simulink model "PVHome"  (R2022b)
settings: Solver=FixedStepDiscrete  StartTime=0.0  StopTime=2  FixedStep=5e-6  RelTol=1e-3
undefined symbols (not defined in the file): Ion, Lithium
libraries: spsSeriesRLCBranchLib x175, spsBreakerLib x103, spsPWMGeneratorDCDCLib x94, spsThyristorLib x78, slpidlib x72, spsIGBTDiodeLib x62, spsThreePhaseVIMeasurementLib x59, spsThreePhaseBreakerLib x45, spsVoltageMeasurementLib x45, spsDiodeLib x39, spsThreePhaseParallelRLCBranchLib x38, spsMosfetLib x32
(part 14 of 16)

== matlab function PVHome/Subsystem2/Centralized System ==
  data: H1_Pv_Breaker output; P_Pv input; Bi_B_Charge_Breaker_Buck output; Bi_B_Charge_Breaker_Boost output; H1_Grid_Breaker output; H1_Grid_Circuit_Breaker output; P_load input; Bi_B_Breaker_Discharge_Boost output; Bi_B_Breaker_Discharge_Buck output; H1_B_Ground_Discharge output; SOCbH1 input; Grid_Energy_Trading_Breaker output; Wind_Breaker_Boost output; P_Wind input; P_Real_Grid input; Wind_Breaker_Buck output; V_PV_1 input; V_Wind input; Wind_Power_Battery_Breaker_Boost output; Wind_Power_Battery_Breaker_Buck output; Battery_Passing_Voltage input; P_PV_2 input; V_PV_2 input; PV_2_Buck_Breaker output; PV_2_Boost_Breaker output
function [H1_Pv_Breaker, Bi_B_Charge_Breaker_Buck,Bi_B_Charge_Breaker_Boost, H1_Grid_Breaker, H1_Grid_Circuit_Breaker,Bi_B_Breaker_Discharge_Boost, Bi_B_Breaker_Discharge_Buck, H1_B_Ground_Discharge, Grid_Energy_Trading_Breaker, Wind_Breaker_Boost, Wind_Breaker_Buck, Wind_Power_Battery_Breaker_Boost, Wind_Power_Battery_Breaker_Buck, PV_2_Buck_Breaker, PV_2_Boost_Breaker] = control_logic(P_Pv, P_load, SOCbH1, P_Wind, P_Real_Grid, V_PV_1, V_Wind, Battery_Passing_Voltage, P_PV_2, V_PV_2)

% Make positive
P_Pv   = abs(P_Pv);
P_load = abs(P_load);
SOCbH1 = abs(SOCbH1);
P_Wind = abs(P_Wind);
V_PV_1 = abs(V_PV_1);
V_Wind = abs(V_Wind);
Battery_Passing_Voltage = abs(Battery_Passing_Voltage);
P_PV_2 = abs(P_PV_2);
V_PV_2 = abs(V_PV_2);

eps = 1;

%% DEFAULT STATES

% DC Ideal Switches (1 = ON) gets closed and power flows when 1
H1_Pv_Breaker = 0;
Bi_B_Charge_Breaker_Buck  = 0;
Bi_B_Charge_Breaker_Boost=0;
Bi_B_Breaker_Discharge_Boost=0;
Bi_B_Breaker_Discharge_Buck=0;
H1_B_Ground_Discharge=0;
Wind_Breaker_Boost=0;
Wind_Breaker_Buck=0;
Wind_Power_Battery_Breaker_Boost=0;
Wind_Power_Battery_Breaker_Buck=0;
PV_2_Buck_Breaker=0;
PV_2_Boost_Breaker=0;

% AC Breakers (0 = CLOSED) gets closed and power flows when 0
H1_Grid_Breaker = 1;  % default OPEN
H1_Grid_Circuit_Breaker = 1;  % default OPEN
Grid_Energy_Trading_Breaker=1; % default open



%% CASE 1: No PV and no Wind
if (P_Pv + P_Wind + P_PV_2) <= eps %eps=0.01 (almost 0)

    % DC OFF
    H1_Pv_Breaker = 0;
    Bi_B_Charge_Breaker_Buck  = 0;
    Bi_B_Breaker_Discharge_Boost=0;
    H1_B_Ground_Discharge=0;
    Bi_B_Breaker_Discharge_Buck=0;
    Wind_Breaker_Boost=0;
    Wind_Breaker_Buck=0;
    Wind_Power_Battery_Breaker_Boost=0;
    Wind_Power_Battery_Breaker_Buck=0;
    PV_2_Boost_Breaker=0;


    % AC CLOSED (use grid)
    H1_Grid_Breaker         = 0;
    H1_Grid_Circuit_Breaker = 1;
    Grid_Energy_Trading_Breaker=1; %energy trading window open


%% CASE 2: PV and wind > Load
elseif (P_Pv + P_Wind + P_PV_2) > P_load

    % Use PV
    H1_Pv_Breaker = 1;
    H1_Grid_Breaker = 1;
    H1_Grid_Circuit_Breaker = 1;

    if (SOCbH1) < 90 % if the value of soc is between is less than 90%, the battery can charge
        
        Bi_B_Breaker_Discharge_Boost=0;
        Bi_B_Breaker_Discharge_Buck=0;
        H1_B_Ground_Discharge=0;
        Grid_Energy_Trading_Breaker=1;
        

        if (V_PV_1 > V_Wind) %boosts up
            Wind_Power_Battery_Breaker_Boost=1;
            Wind_Power_Battery_Breaker_Buck=0;
            Wind_Breaker_Boost=1;
            Wind_Breaker_Buck=0;
            if (Battery_Passing_Voltage)>60
                Bi_B_Charge_Breaker_Buck=1;
                Bi_B_Charge_Breaker_Boost=0;
            elseif (Battery_Passing_Voltage<60)
                Bi_B_Charge_Breaker_Buck=0;
                Bi_B_Charge_Breaker_Boost=1;
            end

        elseif (V_PV_1 < V_Wind)
            Wind_Power_Battery_Breaker_Boost=0;
            Wind_Power_Battery_Breaker_Buck=1;
            Wind_Breaker_Boost=0;
            Wind_Breaker_Buck=1;
        
            if (Battery_Passing_Voltage)>60
                Bi_B_Charge_Breaker_Buck=1;
                Bi_B_Charge_Breaker_Boost=0;
            elseif (Battery_Passing_Voltage)<60
                Bi_B_Charge_Breaker_Buck=0;
                Bi_B_Charge_Breaker_Boost=1;
            end

        
        end 

        elseif (V_PV_2>V_PV_1)
            PV_2_Buck_Breaker=1;
            PV_2_Boost_Breaker=0;
        elseif (V_PV_2<V_PV_1)
            PV_2_Buck_Breaker=0;
            PV_2_Boost_Breaker=1;

        elseif SOCbH1==90
            Bi_B_Charge_Breaker_Boost=0;
            Bi_B_Charge_Breaker_Buck = 0;
            Bi_B_Breaker_Discharge_Boost=0;
            Bi_B_Breaker_Discharge_Buck=0;
            H1_B_Ground_Discharge=0;
            Grid_Energy_Trading_Breaker=0; %the power is sold to grid
        end


%% CASE 3: PV and wind < Load
elseif (P_Pv + P_Wind + P_PV_2) < (P_load) && (H1_Grid_Breaker~=0) %open (1 means open)

    % Use PV
    H1_Pv_Breaker = 1;
    H1_Grid_Circuit_Breaker = 0;
    Grid_Energy_Trading_Breaker=1;      
    Bi_B_Charge_Breaker_Buck=0; %no charging
    Bi_B_Charge_Breaker_Boost=0; %no charging

    if (V_PV_2>V_PV_1)
        PV_2_Buck_Breaker=1;
        PV_2_Boost_Breaker=0;
    elseif (V_PV_2<V_PV_1)
         PV_2_Buck_Breaker=0;
         PV_2_Boost_Breaker=1;
    end

    if (V_PV_1)>60
        Bi_B_Breaker_Discharge_Boost=1;
        Bi_B_Breaker_Discharge_Buck=0;
        H1_B_Ground_Discharge=1;
    elseif(V_PV_1)<60
        Bi_B_Breaker_Discharge_Boost=0;
        Bi_B_Breaker_Discharge_Buck=1;
        H1_B_Ground_Discharge=1;
    end

    if (V_PV_1 > V_Wind) %boosts up
        Wind_Power_Battery_Breaker_Boost=1;
        Wind_Power_Battery_Breaker_Buck=0;
        Wind_Breaker_Boost=1;
        Wind_Breaker_Buck=0;
        
    elseif (V_PV_1 < V_Wind)
        Wind_Power_Battery_Breaker_Boost=0;
        Wind_Power_Battery_Breaker_Buck=1;
        Wind_Breaker_Boost=0;
        Wind_Breaker_Buck=1;
    end 

    
   

           
%% CASE 4:
elseif (P_Pv + P_Wind + P_PV_2) < (P_load) && (H1_Grid_Breaker~=1) %closed (0) (no charging)

        % Use PV
    H1_Pv_Breaker = 1;
    H1_Grid_Circuit_Breaker = 0;
    Grid_Energy_Trading_Breaker=1;      
    Bi_B_Charge_Breaker_Buck=0; %(no charging)
    Bi_B_Charge_Breaker_Boost=0; %(no charging)
    Bi_B_Breaker_Discharge_Boost=0; %(no discharging also)
    Bi_B_Breaker_Discharge_Buck=0; %(no discharging also)
    H1_B_Ground_Discharge=0;

    if (V_PV_2>V_PV_1)
        PV_2_Buck_Breaker=1;
        PV_2_Boost_Breaker=0;
    elseif (V_PV_2<V_PV_1)
         PV_2_Buck_Breaker=0;
         PV_2_Boost_Breaker=1;
    end


    if (V_PV_1 > V_Wind) %boosts up
        Wind_Power_Battery_Breaker_Boost=1;
        Wind_Power_Battery_Breaker_Buck=0;
        Wind_Breaker_Boost=1;
        Wind_Breaker_Buck=0;
        
    elseif (V_PV_1 < V_Wind)
        Wind_Power_Battery_Breaker_Boost=0;
        Wind_Power_Battery_Breaker_Buck=1;
        Wind_Breaker_Boost=0;
        Wind_Breaker_Buck=1;
    end 


%% CASE 5:
elseif (P_Pv + P_Wind+ P_Real_Grid + P_PV_2) < P_Load 
    % Use PV
    H1_Grid_Breaker=0;
    H1_Pv_Breaker = 1;
    H1_Grid_Circuit_Breaker = 0;
    Grid_Energy_Trading_Breaker=1;      
    Bi_B_Charge_Breaker_Buck=0; %(no charging)
    Bi_B_Charge_Breaker_Boost=0; %(no charging)



    %discharging
    if (V_PV_1)>60
        Bi_B_Breaker_Discharge_Boost=1;
        Bi_B_Breaker_Discharge_Buck=0;
        H1_B_Ground_Discharge=1;
    elseif(V_PV_1)<60
        Bi_B_Breaker_Discharge_Boost=0;
        Bi_B_Breaker_Discharge_Buck=1;
        H1_B_Ground_Discharge=1;
    end

    if (V_PV_2>V_PV_1)
        PV_2_Buck_Breaker=1;
        PV_2_Boost_Breaker=0;
    elseif (V_PV_2<V_PV_1)
         PV_2_Buck_Breaker=0;
         PV_2_Boost_Breaker=1;
    end

    if (V_PV_1 > V_Wind) %boosts up
        Wind_Power_Battery_Breaker_Boost=1;
        Wind_Power_Battery_Breaker_Buck=0;
        Wind_Breaker_Boost=1;
        Wind_Breaker_Buck=0;
        
    elseif (V_PV_1 < V_Wind) %bucks down
        Wind_Power_Battery_Breaker_Boost=0;
        Wind_Power_Battery_Breaker_Buck=1;
        Wind_Breaker_Boost=0;
        Wind_Breaker_Buck=1;
    end 

end


end

== matlab function PVHome/Subsystem2/MATLAB Function ==
  data: V_PV input; duty output; I_PV input; deltaD input
function duty = mppt_pno(V_PV, I_PV, deltaD)

persistent prevP prevDuty

if isempty(prevP)
    prevP = 0;
    prevDuty = 0.5;   % Start at 50%
end

% Current PV power
P = V_PV * I_PV;

% Basic P&O
if P > prevP
    prevDuty = prevDuty + deltaD;
else
    prevDuty = prevDuty - deltaD;
end

% Safe duty limits for boost converter
if prevDuty > 0.75
    prevDuty = 0.75;
elseif prevDuty < 0.10
    prevDuty = 0.10;
end

% Update previous power
prevP = P;

% Output duty
duty = prevDuty;

end

== matlab function PVHome/Subsystem2/MATLAB Function1 ==
  data: u input
function export_live_data(u)
% export_live_data  MATLAB Function block that writes 4 signals live into Excel
% Input: u (4-element vector)
% Exact workbook path used: 'V:\IEEE\LIVEdata.xlsx'
%
% Structure preserved: all COM/workspace actions run via evalin('base', ...)

    coder.extrinsic('evalin','assignin','actxserver','datetime','char','warning');

    persistent initialized
    if isempty(initialized)
        initialized = false;
    end

    % Convert inputs to doubles
    a = double(u(1)); b = double(u(2)); c = double(u(3)); d = double(u(4));

    % Use an .xlsx workbook for live UI updates
    excelPath = 'V:\IEEE\LIVEdata.csv';

    % Initialization block executed once (all logic runs inside evalin strings)
    if ~initialized
        % Ensure Excel COM server exists in base workspace and open/create workbook
        evalin('base', [ ...
            'if ~exist(''excelApp'',''var'') || isempty(excelApp), ' ...
                'excelApp = actxserver(''Excel.Application''); excelApp.Visible = true; ' ...
            'end; ' ...
            'if exist(''' excelPath ''',''file'')==2, ' ...
                'wb = excelApp.Workbooks.Open(''' excelPath '''); ws = wb.Worksheets.Item(1); ' ...
            'else, ' ...
                'wb = excelApp.Workbooks.Add; ws = wb.Worksheets.Item(1); ' ...
                'ws.Range(''A1'').Value = ''Timestamp''; ws.Range(''B1'').Value = ''Signal1''; ' ...
                'ws.Range(''C1'').Value = ''Signal2''; ws.Range(''D1'').Value = ''Signal3''; ' ...
                'ws.Range(''E1'').Value = ''Signal4''; wb.SaveAs(''' excelPath '''); ' ...
            'end; ' ...
            'if ~exist(''excelRow'',''var'') || isempty(excelRow), ur = ws.UsedRange; excelRow = double(ur.Rows.Count) + 1; end;']);

        initialized = true;
    end

    % Create timestamp string using datetime (host MATLAB)
    ts = char(datetime('now', 'Format', 'yyyy-MM-dd HH:mm:ss.SSS'));

    % Pass values into base workspace temporary variables (RHS only)
    assignin('base', 'tmp_ts', ts);
    assignin('base', 'tmp_a', a);
    assignin('base', 'tmp_b', b);
    assignin('base', 'tmp_c', c);
    assignin('base', 'tmp_d', d);

    % Perform the worksheet write and force Excel UI update (all inside evalin)
    % Note: r is the row written; we save, increment excelRow, then force repaint and scroll.
    evalin('base', [ ...
        'r = excelRow; ' ...
        'ws.Range([''A'' num2str(r)]).Value = tmp_ts; ' ...
        'ws.Range([''B'' num2str(r)]).Value = tmp_a; ' ...
        'ws.Range([''C'' num2str(r)]).Value = tmp_b; ' ...
        'ws.Range([''D'' num2str(r)]).Value = tmp_c; ' ...
        'ws.Range([''E'' num2str(r)]).Value = tmp_d; ' ...
        'wb.Save; ' ...
        'excelRow = r + 1; ' ...
        'try, excelApp.ScreenUpdating = true; excelApp.Calculate; ' ...
             'if ~isempty(excelApp.ActiveWindow), excelApp.ActiveWindow.ScrollRow = r; end; ' ...
             'pause(0.02); ' ...
        'end;']);

end

== matlab function PVHome/Subsystem3/Centralized System ==
  data: H1_Pv_Breaker output; P_Pv input; Bi_B_Charge_Breaker_Buck output; Bi_B_Charge_Breaker_Boost output; H1_Grid_Breaker output; H1_Grid_Circuit_Breaker output; P_load input; Bi_B_Breaker_Discharge_Boost output; Bi_B_Breaker_Discharge_Buck output; H1_B_Ground_Discharge output; SOCbH1 input; Grid_Energy_Trading_Breaker output; Wind_Breaker_Boost output; P_Wind input; P_Real_Grid input; Wind_Breaker_Buck output; V_PV_1 input; V_Wind input; Wind_Power_Battery_Breaker_Boost output; Wind_Power_Battery_Breaker_Buck output; Battery_Passing_Voltage input; P1_C1 output
function [H1_Pv_Breaker, Bi_B_Charge_Breaker_Buck,Bi_B_Charge_Breaker_Boost, H1_Grid_Breaker, H1_Grid_Circuit_Breaker,Bi_B_Breaker_Discharge_Boost, Bi_B_Breaker_Discharge_Buck, H1_B_Ground_Discharge, Grid_Energy_Trading_Breaker, Wind_Breaker_Boost, Wind_Breaker_Buck, Wind_Power_Battery_Breaker_Boost, Wind_Power_Battery_Breaker_Buck, P1_C1] = control_logic(P_Pv, P_load, SOCbH1, P_Wind, P_Real_Grid, V_PV_1, V_Wind, Battery_Passing_Voltage)

% Make positive
P_Pv   = abs(P_Pv);
P_load = abs(P_load);
SOCbH1 = abs(SOCbH1);
P_Wind = abs(P_Wind);
V_PV_1 = abs(V_PV_1);
V_Wind = abs(V_Wind);
Battery_Passing_Voltage = abs(Battery_Passing_Voltage);

eps = 1;

%% DEFAULT STATES

% DC Ideal Switches (1 = ON)
H1_Pv_Breaker = 0;
Bi_B_Charge_Breaker_Buck  = 0;
Bi_B_Charge_Breaker_Boost=0;
Bi_B_Breaker_Discharge_Boost=0;
Bi_B_Breaker_Discharge_Buck=0;
H1_B_Ground_Discharge=0;
Wind_Breaker_Boost=0;
Wind_Breaker_Buck=0;
Wind_Power_Battery_Breaker_Boost=0;
Wind_Power_Battery_Breaker_Buck=0;
P1_C1=0;

% AC Breakers (0 = CLOSED)
H1_Grid_Breaker = 1;  % default OPEN
H1_Grid_Circuit_Breaker = 1;  % default OPEN
Grid_Energy_Trading_Breaker=1; % default open



%% CASE 1: No PV and no Wind
if (P_Pv+ P_Wind) <= eps %eps=0.01 (almost 0)

    % DC OFF
    H1_Pv_Breaker = 0;
    Bi_B_Charge_Breaker_Buck  = 0;
    Bi_B_Breaker_Discharge_Boost=0;
    H1_B_Ground_Discharge=0;
    Bi_B_Breaker_Discharge_Buck=0;
    Wind_Breaker_Boost=0;
    Wind_Breaker_Buck=0;
    Wind_Power_Battery_Breaker_Boost=0;
    Wind_Power_Battery_Breaker_Buck=0;
    P1_C1=0;


    % AC CLOSED (use grid)
    H1_Grid_Breaker         = 0;
    H1_Grid_Circuit_Breaker = 1;
    Grid_Energy_Trading_Breaker=1; %energy trading window open


%% CASE 2: PV and wind > Load
elseif (P_Pv + P_Wind) > P_load

    % Use PV
    H1_Pv_Breaker = 1;
    H1_Grid_Breaker = 1;
    H1_Grid_Circuit_Breaker = 1;

    if (SOCbH1) < 90 % if the value of soc is between is less than 90%, the battery can charge
        
        Bi_B_Breaker_Discharge_Boost=0;
        Bi_B_Breaker_Discharge_Buck=0;
        H1_B_Ground_Discharge=0;
        Grid_Energy_Trading_Breaker=1;
        P1_C1=0;        

        if (V_PV_1 > V_Wind) %boosts up
            Wind_Power_Battery_Breaker_Boost=1;
            Wind_Power_Battery_Breaker_Buck=0;
            Wind_Breaker_Boost=1;
            Wind_Breaker_Buck=0;
            if (Battery_Passing_Voltage)>60
                Bi_B_Charge_Breaker_Buck=1;
                Bi_B_Charge_Breaker_Boost=0;
            elseif (Battery_Passing_Voltage<60)
                Bi_B_Charge_Breaker_Buck=0;
                Bi_B_Charge_Breaker_Boost=1;
            end

        elseif (V_PV_1 < V_Wind)
            Wind_Power_Battery_Breaker_Boost=0;
            Wind_Power_Battery_Breaker_Buck=1;
            Wind_Breaker_Boost=0;
            Wind_Breaker_Buck=1;
        
            if (Battery_Passing_Voltage)>60
                Bi_B_Charge_Breaker_Buck=1;
                Bi_B_Charge_Breaker_Boost=0;
            elseif (Battery_Passing_Voltage)<60
                Bi_B_Charge_Breaker_Buck=0;
                Bi_B_Charge_Breaker_Boost=1;
            end
        
        end

    elseif SOCbH1==90
        Bi_B_Charge_Breaker_Boost=0;
        Bi_B_Charge_Breaker_Buck = 0;
        Bi_B_Breaker_Discharge_Boost=0;
        Bi_B_Breaker_Discharge_Buck=0;
        H1_B_Ground_Discharge=0;
        Grid_Energy_Trading_Breaker=0; %the power is sold to grid
        P1_C1=1; %the power is sold to C1

        if (V_PV_1 > V_Wind) %boosts up
        Wind_Power_Battery_Breaker_Boost=1;
        Wind_Power_Battery_Breaker_Buck=0;
        Wind_Breaker_Boost=1;
        Wind_Breaker_Buck=0;
        if (Battery_Passing_Voltage)>60
            Bi_B_Charge_Breaker_Buck=1;
            Bi_B_Charge_Breaker_Boost=0;
        elseif (Battery_Passing_Voltage<60)
            Bi_B_Charge_Breaker_Buck=0;
            Bi_B_Charge_Breaker_Boost=1;
        end

    elseif (V_PV_1 < V_Wind)
        Wind_Power_Battery_Breaker_Boost=0;
        Wind_Power_Battery_Breaker_Buck=1;
        Wind_Breaker_Boost=0;
        Wind_Breaker_Buck=1;
        
        if (Battery_Passing_Voltage)>60
            Bi_B_Charge_Breaker_Buck=1;
            Bi_B_Charge_Breaker_Boost=0;
        elseif (Battery_Passing_Voltage)<60
            Bi_B_Charge_Breaker_Buck=0;
            Bi_B_Charge_Breaker_Boost=1;
        end
        end
    end



%% CASE 3: PV and wind < Load
elseif (P_Pv + P_Wind) < (P_load) && (H1_Grid_Breaker~=0) %open (1 means open)

    % Use PV
    H1_Pv_Breaker = 1;
    H1_Grid_Circuit_Breaker = 0;
    Grid_Energy_Trading_Breaker=1;      
    Bi_B_Charge_Breaker_Buck=0; %no charging
    Bi_B_Charge_Breaker_Boost=0; %no charging
    P1_C1=0;


    if (V_PV_1)>60
        Bi_B_Breaker_Discharge_Boost=1;
        Bi_B_Breaker_Discharge_Buck=0;
        H1_B_Ground_Discharge=1;
    elseif(V_PV_1)<60
        Bi_B_Breaker_Discharge_Boost=0;
        Bi_B_Breaker_Discharge_Buck=1;
        H1_B_Ground_Discharge=1;
    end

    if (V_PV_1 > V_Wind) %boosts up
        Wind_Power_Battery_Breaker_Boost=1;
        Wind_Power_Battery_Breaker_Buck=0;
        Wind_Breaker_Boost=1;
        Wind_Breaker_Buck=0;
        
    elseif (V_PV_1 < V_Wind)
        Wind_Power_Battery_Breaker_Boost=0;
        Wind_Power_Battery_Breaker_Buck=1;
        Wind_Breaker_Boost=0;
        Wind_Breaker_Buck=1;
    end 

    
   

           
%% CASE 4:
elseif (P_Pv + P_Wind) < (P_load) && (H1_Grid_Breaker~=1) %closed (0) (no charging)

        % Use PV
    H1_Pv_Breaker = 1;
    H1_Grid_Circuit_Breaker = 0;
    Grid_Energy_Trading_Breaker=1;      
    Bi_B_Charge_Breaker_Buck=0; %(no charging)
    Bi_B_Charge_Breaker_Boost=0; %(no charging)
    Bi_B_Breaker_Discharge_Boost=0;
    Bi_B_Breaker_Discharge_Buck=0;
    H1_B_Ground_Discharge=0;
    P1_C1=0;


    if (V_PV_1 > V_Wind) %boosts up
        Wind_Power_Battery_Breaker_Boost=1;
        Wind_Power_Battery_Breaker_Buck=0;
        Wind_Breaker_Boost=1;
        Wind_Breaker_Buck=0;
        
    elseif (V_PV_1 < V_Wind)
        Wind_Power_Battery_Breaker_Boost=0;
        Wind_Power_Battery_Breaker_Buck=1;
        Wind_Breaker_Boost=0;
        Wind_Breaker_Buck=1;
    end 


%% CASE 5:
elseif (P_Pv + P_Wind+ P_Real_Grid) < P_Load 
    % Use PV
    H1_Grid_Breaker=0;
    H1_Pv_Breaker = 1;
    H1_Grid_Circuit_Breaker = 0;
    Grid_Energy_Trading_Breaker=1;      
    Bi_B_Charge_Breaker_Buck=0; %(no charging)
    Bi_B_Charge_Breaker_Boost=0; %(no charging)
    P1_C1=0;

    %discharging
    if (V_PV_1)>60
        Bi_B_Breaker_Discharge_Boost=1;
        Bi_B_Breaker_Discharge_Buck=0;
        H1_B_Ground_Discharge=1;
    elseif(V_PV_1)<60
        Bi_B_Breaker_Discharge_Boost=0;
        Bi_B_Breaker_Discharge_Buck=1;
        H1_B_Ground_Discharge=1;
    end

    if (V_PV_1 > V_Wind) %boosts up
        Wind_Power_Battery_Breaker_Boost=1;
        Wind_Power_Battery_Breaker_Buck=0;
        Wind_Breaker_Boost=1;
        Wind_Breaker_Buck=0;
        
    elseif (V_PV_1 < V_Wind) %bucks down
        Wind_Power_Battery_Breaker_Boost=0;
        Wind_Power_Battery_Breaker_Buck=1;
        Wind_Breaker_Boost=0;
        Wind_Breaker_Buck=1;
    end 

end


end

== matlab function PVHome/Subsystem3/MATLAB Function ==
  data: V_PV input; duty output; I_PV input; deltaD input
function duty = mppt_pno(V_PV, I_PV, deltaD)

persistent prevP prevDuty

if isempty(prevP)
    prevP = 0;
    prevDuty = 0.5;   % Start at 50%
end

% Current PV power
P = V_PV * I_PV;

% Basic P&O
if P > prevP
    prevDuty = prevDuty + deltaD;
else
    prevDuty = prevDuty - deltaD;
end

% Safe duty limits for boost converter
if prevDuty > 0.75
    prevDuty = 0.75;
elseif prevDuty < 0.10
    prevDuty = 0.10;
end

% Update previous power
prevP = P;

% Output duty
duty = prevDuty;

end

== matlab function PVHome/Subsystem3/MATLAB Function1 ==
  data: u input
function export_live_data(u)
% export_live_data  MATLAB Function block that writes 4 signals live into Excel
% Input: u (4-element vector)
% Exact workbook path used: 'V:\IEEE\LIVEdata.xlsx'
%
% Structure preserved: all COM/workspace actions run via evalin('base', ...)

    coder.extrinsic('evalin','assignin','actxserver','datetime','char','warning');

    persistent initialized
    if isempty(initialized)
        initialized = false;
    end

    % Convert inputs to doubles
    a = double(u(1)); b = double(u(2)); c = double(u(3)); d = double(u(4));

    % Use an .xlsx workbook for live UI updates
    excelPath = 'V:\IEEE\LIVEdata.csv';

    % Initialization block executed once (all logic runs inside evalin strings)
    if ~initialized
        % Ensure Excel COM server exists in base workspace and open/create workbook
        evalin('base', [ ...
            'if ~exist(''excelApp'',''var'') || isempty(excelApp), ' ...
                'excelApp = actxserver(''Excel.Application''); excelApp.Visible = true; ' ...
            'end; ' ...
            'if exist(''' excelPath ''',''file'')==2, ' ...
                'wb = excelApp.Workbooks.Open(''' excelPath '''); ws = wb.Worksheets.Item(1); ' ...
            'else, ' ...
                'wb = excelApp.Workbooks.Add; ws = wb.Worksheets.Item(1); ' ...
                'ws.Range(''A1'').Value = ''Timestamp''; ws.Range(''B1'').Value = ''Signal1''; ' ...
                'ws.Range(''C1'').Value = ''Signal2''; ws.Range(''D1'').Value = ''Signal3''; ' ...
                'ws.Range(''E1'').Value = ''Signal4''; wb.SaveAs(''' excelPath '''); ' ...
            'end; ' ...
            'if ~exist(''excelRow'',''var'') || isempty(excelRow), ur = ws.UsedRange; excelRow = double(ur.Rows.Count) + 1; end;']);

        initialized = true;
    end

    % Create timestamp string using datetime (host MATLAB)
    ts = char(datetime('now', 'Format', 'yyyy-MM-dd HH:mm:ss.SSS'));

    % Pass values into base workspace temporary variables (RHS only)
    assignin('base', 'tmp_ts', ts);
    assignin('base', 'tmp_a', a);
    assignin('base', 'tmp_b', b);
    assignin('base', 'tmp_c', c);
    assignin('base', 'tmp_d', d);

    % Perform the worksheet write and force Excel UI update (all inside evalin)
    % Note: r is the row written; we save, increment excelRow, then force repaint and scroll.
    evalin('base', [ ...
        'r = excelRow; ' ...
        'ws.Range([''A'' num2str(r)]).Value = tmp_ts; ' ...
        'ws.Range([''B'' num2str(r)]).Value = tmp_a; ' ...
        'ws.Range([''C'' num2str(r)]).Value = tmp_b; ' ...
        'ws.Range([''D'' num2str(r)]).Value = tmp_c; ' ...
        'ws.Range([''E'' num2str(r)]).Value = tmp_d; ' ...
        'wb.Save; ' ...
        'excelRow = r + 1; ' ...
        'try, excelApp.ScreenUpdating = true; excelApp.Calculate; ' ...
             'if ~isempty(excelApp.ActiveWindow), excelApp.ActiveWindow.ScrollRow = r; end; ' ...
             'pause(0.02); ' ...
        'end;']);

end

== matlab function PVHome/Subsystem4/Centralized System ==
  data: H1_Pv_Breaker output; P_Pv input; Bi_B_Charge_Breaker_Buck output; Bi_B_Charge_Breaker_Boost output; H1_Grid_Breaker output; H1_Grid_Circuit_Breaker output; P_load input; Bi_B_Breaker_Discharge_Boost output; Bi_B_Breaker_Discharge_Buck output; H1_B_Ground_Discharge output; SOCbH1 input; Grid_Energy_Trading_Breaker output; Wind_Breaker_Boost output; P_Wind input; P_Real_Grid input; Wind_Breaker_Buck output; V_PV_1 input; V_Wind input; Wind_Power_Battery_Breaker_Boost output; Wind_Power_Battery_Breaker_Buck output; Battery_Passing_Voltage input; P1_C1 output
function [H1_Pv_Breaker, Bi_B_Charge_Breaker_Buck,Bi_B_Charge_Breaker_Boost, H1_Grid_Breaker, H1_Grid_Circuit_Breaker,Bi_B_Breaker_Discharge_Boost, Bi_B_Breaker_Discharge_Buck, H1_B_Ground_Discharge, Grid_Energy_Trading_Breaker, Wind_Breaker_Boost, Wind_Breaker_Buck, Wind_Power_Battery_Breaker_Boost, Wind_Power_Battery_Breaker_Buck, P1_C1] = control_logic(P_Pv, P_load, SOCbH1, P_Wind, P_Real_Grid, V_PV_1, V_Wind, Battery_Passing_Voltage)

% Make positive
P_Pv   = abs(P_Pv);
P_load = abs(P_load);
SOCbH1 = abs(SOCbH1);
P_Wind = abs(P_Wind);
V_PV_1 = abs(V_PV_1);
V_Wind = abs(V_Wind);
Battery_Passing_Voltage = abs(Battery_Passing_Voltage);

eps = 1;

%% DEFAULT STATES

% DC Ideal Switches (1 = ON)
H1_Pv_Breaker = 0;
Bi_B_Charge_Breaker_Buck  = 0;
Bi_B_Charge_Breaker_Boost=0;
Bi_B_Breaker_Discharge_Boost=0;
Bi_B_Breaker_Discharge_Buck=0;
H1_B_Ground_Discharge=0;
Wind_Breaker_Boost=0;
Wind_Breaker_Buck=0;
Wind_Power_Battery_Breaker_Boost=0;
Wind_Power_Battery_Breaker_Buck=0;
P1_C1=0;

% AC Breakers (0 = CLOSED)
H1_Grid_Breaker = 1;  % default OPEN
H1_Grid_Circuit_Breaker = 1;  % default OPEN
Grid_Energy_Trading_Breaker=1; % default open



%% CASE 1: No PV and no Wind
if (P_Pv+ P_Wind) <= eps %eps=0.01 (almost 0)

    % DC OFF
    H1_Pv_Breaker = 0;
    Bi_B_Charge_Breaker_Buck  = 0;
    Bi_B_Breaker_Discharge_Boost=0;
    H1_B_Ground_Discharge=0;
    Bi_B_Breaker_Discharge_Buck=0;
    Wind_Breaker_Boost=0;
    Wind_Breaker_Buck=0;
    Wind_Power_Battery_Breaker_Boost=0;
    Wind_Power_Battery_Breaker_Buck=0;
    P1_C1=0;


    % AC CLOSED (use grid)
    H1_Grid_Breaker         = 0;
    H1_Grid_Circuit_Breaker = 1;
    Grid_Energy_Trading_Breaker=1; %energy trading window open


%% CASE 2: PV and wind > Load
elseif (P_Pv + P_Wind) > P_load

    % Use PV
    H1_Pv_Breaker = 1;
    H1_Grid_Breaker = 1;
    H1_Grid_Circuit_Breaker = 1;

    if (SOCbH1) < 90 % if the value of soc is between is less than 90%, the battery can charge
        
        Bi_B_Breaker_Discharge_Boost=0;
        Bi_B_Breaker_Discharge_Buck=0;
        H1_B_Ground_Discharge=0;
        Grid_Energy_Trading_Breaker=1;
        P1_C1=0;        

        if (V_PV_1 > V_Wind) %boosts up
            Wind_Power_Battery_Breaker_Boost=1;
            Wind_Power_Battery_Breaker_Buck=0;
            Wind_Breaker_Boost=1;
            Wind_Breaker_Buck=0;
            if (Battery_Passing_Voltage)>60
                Bi_B_Charge_Breaker_Buck=1;
                Bi_B_Charge_Breaker_Boost=0;
            elseif (Battery_Passing_Voltage<60)
                Bi_B_Charge_Breaker_Buck=0;
                Bi_B_Charge_Breaker_Boost=1;
            end

        elseif (V_PV_1 < V_Wind)
            Wind_Power_Battery_Breaker_Boost=0;
            Wind_Power_Battery_Breaker_Buck=1;
            Wind_Breaker_Boost=0;
            Wind_Breaker_Buck=1;
        
            if (Battery_Passing_Voltage)>60
                Bi_B_Charge_Breaker_Buck=1;
                Bi_B_Charge_Breaker_Boost=0;
            elseif (Battery_Passing_Voltage)<60
                Bi_B_Charge_Breaker_Buck=0;
                Bi_B_Charge_Breaker_Boost=1;
            end
        
        end

    elseif SOCbH1==90
        Bi_B_Charge_Breaker_Boost=0;
        Bi_B_Charge_Breaker_Buck = 0;
        Bi_B_Breaker_Discharge_Boost=0;
        Bi_B_Breaker_Discharge_Buck=0;
        H1_B_Ground_Discharge=0;
        Grid_Energy_Trading_Breaker=0; %the power is sold to grid
        P1_C1=1; %the power is sold to C1

        if (V_PV_1 > V_Wind) %boosts up
        Wind_Power_Battery_Breaker_Boost=1;
        Wind_Power_Battery_Breaker_Buck=0;
        Wind_Breaker_Boost=1;
        Wind_Breaker_Buck=0;
        if (Battery_Passing_Voltage)>60
            Bi_B_Charge_Breaker_Buck=1;
            Bi_B_Charge_Breaker_Boost=0;
        elseif (Battery_Passing_Voltage<60)
            Bi_B_Charge_Breaker_Buck=0;
            Bi_B_Charge_Breaker_Boost=1;
        end

    elseif (V_PV_1 < V_Wind)
        Wind_Power_Battery_Breaker_Boost=0;
        Wind_Power_Battery_Breaker_Buck=1;
        Wind_Breaker_Boost=0;
        Wind_Breaker_Buck=1;
        
        if (Battery_Passing_Voltage)>60
            Bi_B_Charge_Breaker_Buck=1;
            Bi_B_Charge_Breaker_Boost=0;
        elseif (Battery_Passing_Voltage)<60
            Bi_B_Charge_Breaker_Buck=0;
            Bi_B_Charge_Breaker_Boost=1;
        end
        end
    end



%% CASE 3: PV and wind < Load
elseif (P_Pv + P_Wind) < (P_load) && (H1_Grid_Breaker~=0) %open (1 means open)

    % Use PV
    H1_Pv_Breaker = 1;
    H1_Grid_Circuit_Breaker = 0;
    Grid_Energy_Trading_Breaker=1;      
    Bi_B_Charge_Breaker_Buck=0; %no charging
    Bi_B_Charge_Breaker_Boost=0; %no charging
    P1_C1=0;


    if (V_PV_1)>60
        Bi_B_Breaker_Discharge_Boost=1;
        Bi_B_Breaker_Discharge_Buck=0;
        H1_B_Ground_Discharge=1;
    elseif(V_PV_1)<60
        Bi_B_Breaker_Discharge_Boost=0;
        Bi_B_Breaker_Discharge_Buck=1;
        H1_B_Ground_Discharge=1;
    end

    if (V_PV_1 > V_Wind) %boosts up
        Wind_Power_Battery_Breaker_Boost=1;
        Wind_Power_Battery_Breaker_Buck=0;
        Wind_Breaker_Boost=1;
        Wind_Breaker_Buck=0;
        
    elseif (V_PV_1 < V_Wind)
        Wind_Power_Battery_Breaker_Boost=0;
        Wind_Power_Battery_Breaker_Buck=1;
        Wind_Breaker_Boost=0;
        Wind_Breaker_Buck=1;
    end 

    
   

           
%% CASE 4:
elseif (P_Pv + P_Wind) < (P_load) && (H1_Grid_Breaker~=1) %closed (0) (no charging)

        % Use PV
    H1_Pv_Breaker = 1;
    H1_Grid_Circuit_Breaker = 0;
    Grid_Energy_Trading_Breaker=1;      
    Bi_B_Charge_Breaker_Buck=0; %(no charging)
    Bi_B_Charge_Breaker_Boost=0; %(no charging)
    Bi_B_Breaker_Discharge_Boost=0;
    Bi_B_Breaker_Discharge_Buck=0;
    H1_B_Ground_Discharge=0;
    P1_C1=0;


    if (V_PV_1 > V_Wind) %boosts up
        Wind_Power_Battery_Breaker_Boost=1;
        Wind_Power_Battery_Breaker_Buck=0;
        Wind_Breaker_Boost=1;
        Wind_Breaker_Buck=0;
        
    elseif (V_PV_1 < V_Wind)
        Wind_Power_Battery_Breaker_Boost=0;
        Wind_Power_Battery_Breaker_Buck=1;
        Wind_Breaker_Boost=0;
        Wind_Breaker_Buck=1;
    end 


%% CASE 5:
elseif (P_Pv + P_Wind+ P_Real_Grid) < P_Load 
    % Use PV
    H1_Grid_Breaker=0;
    H1_Pv_Breaker = 1;
    H1_Grid_Circuit_Breaker = 0;
    Grid_Energy_Trading_Breaker=1;      
    Bi_B_Charge_Breaker_Buck=0; %(no charging)
    Bi_B_Charge_Breaker_Boost=0; %(no charging)
    P1_C1=0;

    %discharging
    if (V_PV_1)>60
        Bi_B_Breaker_Discharge_Boost=1;
        Bi_B_Breaker_Discharge_Buck=0;
        H1_B_Ground_Discharge=1;
    elseif(V_PV_1)<60
        Bi_B_Breaker_Discharge_Boost=0;
        Bi_B_Breaker_Discharge_Buck=1;
        H1_B_Ground_Discharge=1;
    end

    if (V_PV_1 > V_Wind) %boosts up
        Wind_Power_Battery_Breaker_Boost=1;
        Wind_Power_Battery_Breaker_Buck=0;
        Wind_Breaker_Boost=1;
        Wind_Breaker_Buck=0;
        
    elseif (V_PV_1 < V_Wind) %bucks down
        Wind_Power_Battery_Breaker_Boost=0;
        Wind_Power_Battery_Breaker_Buck=1;
        Wind_Breaker_Boost=0;
        Wind_Breaker_Buck=1;
    end 

end


end

== matlab function PVHome/Subsystem4/MATLAB Function ==
  data: V_PV input; duty output; I_PV input; deltaD input
function duty = mppt_pno(V_PV, I_PV, deltaD)

persistent prevP prevDuty

if isempty(prevP)
    prevP = 0;
    prevDuty = 0.5;   % Start at 50%
end

% Current PV power
P = V_PV * I_PV;

% Basic P&O
if P > prevP
    prevDuty = prevDuty + deltaD;
else
    prevDuty = prevDuty - deltaD;
end

% Safe duty limits for boost converter
if prevDuty > 0.75
    prevDuty = 0.75;
elseif prevDuty < 0.10
    prevDuty = 0.10;
end

% Update previous power
prevP = P;

% Output duty
duty = prevDuty;

end

== matlab function PVHome/Subsystem4/MATLAB Function1 ==
  data: u input
function export_live_data(u)
% export_live_data  MATLAB Function block that writes 4 signals live into Excel
% Input: u (4-element vector)
% Exact workbook path used: 'V:\IEEE\LIVEdata.xlsx'
%
% Structure preserved: all COM/workspace actions run via evalin('base', ...)

    coder.extrinsic('evalin','assignin','actxserver','datetime','char','warning');

    persistent initialized
    if isempty(initialized)
        initialized = false;
    end

    % Convert inputs to doubles
    a = double(u(1)); b = double(u(2)); c = double(u(3)); d = double(u(4));

    % Use an .xlsx workbook for live UI updates
    excelPath = 'V:\IEEE\LIVEdata.csv';

    % Initialization block executed once (all logic runs inside evalin strings)
    if ~initialized
        % Ensure Excel COM server exists in base workspace and open/create workbook
        evalin('base', [ ...
            'if ~exist(''excelApp'',''var'') || isempty(excelApp), ' ...
                'excelApp = actxserver(''Excel.Application''); excelApp.Visible = true; ' ...
            'end; ' ...
            'if exist(''' excelPath ''',''file'')==2, ' ...
                'wb = excelApp.Workbooks.Open(''' excelPath '''); ws = wb.Worksheets.Item(1); ' ...
            'else, ' ...
                'wb = excelApp.Workbooks.Add; ws = wb.Worksheets.Item(1); ' ...
                'ws.Range(''A1'').Value = ''Timestamp''; ws.Range(''B1'').Value = ''Signal1''; ' ...
                'ws.Range(''C1'').Value = ''Signal2''; ws.Range(''D1'').Value = ''Signal3''; ' ...
                'ws.Range(''E1'').Value = ''Signal4''; wb.SaveAs(''' excelPath '''); ' ...
            'end; ' ...
            'if ~exist(''excelRow'',''var'') || isempty(excelRow), ur = ws.UsedRange; excelRow = double(ur.Rows.Count) + 1; end;']);

        initialized = true;
    end

    % Create timestamp string using datetime (host MATLAB)
    ts = char(datetime('now', 'Format', 'yyyy-MM-dd HH:mm:ss.SSS'));

    % Pass values into base workspace temporary variables (RHS only)
    assignin('base', 'tmp_ts', ts);
    assignin('base', 'tmp_a', a);
    assignin('base', 'tmp_b', b);
    assignin('base', 'tmp_c', c);
    assignin('base', 'tmp_d', d);

    % Perform the worksheet write and force Excel UI update (all inside evalin)
    % Note: r is the row written; we save, increment excelRow, then force repaint and scroll.
    evalin('base', [ ...
        'r = excelRow; ' ...
        'ws.Range([''A'' num2str(r)]).Value = tmp_ts; ' ...
        'ws.Range([''B'' num2str(r)]).Value = tmp_a; ' ...
        'ws.Range([''C'' num2str(r)]).Value = tmp_b; ' ...
        'ws.Range([''D'' num2str(r)]).Value = tmp_c; ' ...
        'ws.Range([''E'' num2str(r)]).Value = tmp_d; ' ...
        'wb.Save; ' ...
        'excelRow = r + 1; ' ...
        'try, excelApp.ScreenUpdating = true; excelApp.Calculate; ' ...
             'if ~isempty(excelApp.ActiveWindow), excelApp.ActiveWindow.ScrollRow = r; end; ' ...
             'pause(0.02); ' ...
        'end;']);

end

== matlab function PVHome/Subsystem5/Centralized System ==
  data: H1_Pv_Breaker output; P_Pv input; Bi_B_Charge_Breaker_Buck output; Bi_B_Charge_Breaker_Boost output; H1_Grid_Breaker output; H1_Grid_Circuit_Breaker output; P_load input; Bi_B_Breaker_Discharge_Boost output; Bi_B_Breaker_Discharge_Buck output; H1_B_Ground_Discharge output; SOCbH1 input; Grid_Energy_Trading_Breaker output; Wind_Breaker_Boost output; P_Wind input; P_Real_Grid input; Wind_Breaker_Buck output; V_PV_1 input; V_Wind input; Wind_Power_Battery_Breaker_Boost output; Wind_Power_Battery_Breaker_Buck output; Battery_Passing_Voltage input; P1_C1 output
function [H1_Pv_Breaker, Bi_B_Charge_Breaker_Buck,Bi_B_Charge_Breaker_Boost, H1_Grid_Breaker, H1_Grid_Circuit_Breaker,Bi_B_Breaker_Discharge_Boost, Bi_B_Breaker_Discharge_Buck, H1_B_Ground_Discharge, Grid_Energy_Trading_Breaker, Wind_Breaker_Boost, Wind_Breaker_Buck, Wind_Power_Battery_Breaker_Boost, Wind_Power_Battery_Breaker_Buck, P1_C1] = control_logic(P_Pv, P_load, SOCbH1, P_Wind, P_Real_Grid, V_PV_1, V_Wind, Battery_Passing_Voltage)

% Make positive
P_Pv   = abs(P_Pv);
P_load = abs(P_load);
SOCbH1 = abs(SOCbH1);
P_Wind = abs(P_Wind);
V_PV_1 = abs(V_PV_1);
V_Wind = abs(V_Wind);
Battery_Passing_Voltage = abs(Battery_Passing_Voltage);

eps = 1;

%% DEFAULT STATES

% DC Ideal Switches (1 = ON)
H1_Pv_Breaker = 0;
Bi_B_Charge_Breaker_Buck  = 0;
Bi_B_Charge_Breaker_Boost=0;
Bi_B_Breaker_Discharge_Boost=0;
Bi_B_Breaker_Discharge_Buck=0;
H1_B_Ground_Discharge=0;
Wind_Breaker_Boost=0;
Wind_Breaker_Buck=0;
Wind_Power_Battery_Breaker_Boost=0;
Wind_Power_Battery_Breaker_Buck=0;
P1_C1=0;

% AC Breakers (0 = CLOSED)
H1_Grid_Breaker = 1;  % default OPEN
H1_Grid_Circuit_Breaker = 1;  % default OPEN
Grid_Energy_Trading_Breaker=1; % default open



%% CASE 1: No PV and no Wind
if (P_Pv+ P_Wind) <= eps %eps=0.01 (almost 0)

    % DC OFF
    H1_Pv_Breaker = 0;
    Bi_B_Charge_Breaker_Buck  = 0;
    Bi_B_Breaker_Discharge_Boost=0;
    H1_B_Ground_Discharge=0;
    Bi_B_Breaker_Discharge_Buck=0;
    Wind_Breaker_Boost=0;
    Wind_Breaker_Buck=0;
    Wind_Power_Battery_Breaker_Boost=0;
    Wind_Power_Battery_Breaker_Buck=0;
    P1_C1=0;


    % AC CLOSED (use grid)
    H1_Grid_Breaker         = 0;
    H1_Grid_Circuit_Breaker = 1;
    Grid_Energy_Trading_Breaker=1; %energy trading window open


%% CASE 2: PV and wind > Load
elseif (P_Pv + P_Wind) > P_load

    % Use PV
    H1_Pv_Breaker = 1;
    H1_Grid_Breaker = 1;
    H1_Grid_Circuit_Breaker = 1;

    if (SOCbH1) < 90 % if the value of soc is between is less than 90%, the battery can charge
        
        Bi_B_Breaker_Discharge_Boost=0;
        Bi_B_Breaker_Discharge_Buck=0;
        H1_B_Ground_Discharge=0;
        Grid_Energy_Trading_Breaker=1;
        P1_C1=0;        

        if (V_PV_1 > V_Wind) %boosts up
            Wind_Power_Battery_Breaker_Boost=1;
            Wind_Power_Battery_Breaker_Buck=0;
            Wind_Breaker_Boost=1;
            Wind_Breaker_Buck=0;
            if (Battery_Passing_Voltage)>60
                Bi_B_Charge_Breaker_Buck=1;
                Bi_B_Charge_Breaker_Boost=0;
            elseif (Battery_Passing_Voltage<60)
                Bi_B_Charge_Breaker_Buck=0;
                Bi_B_Charge_Breaker_Boost=1;
            end

        elseif (V_PV_1 < V_Wind)
            Wind_Power_Battery_Breaker_Boost=0;
            Wind_Power_Battery_Breaker_Buck=1;
            Wind_Breaker_Boost=0;
            Wind_Breaker_Buck=1;
        
            if (Battery_Passing_Voltage)>60
                Bi_B_Charge_Breaker_Buck=1;
                Bi_B_Charge_Breaker_Boost=0;
            elseif (Battery_Passing_Voltage)<60
                Bi_B_Charge_Breaker_Buck=0;
                Bi_B_Charge_Breaker_Boost=1;
            end
        
        end

    elseif SOCbH1==90
        Bi_B_Charge_Breaker_Boost=0;
        Bi_B_Charge_Breaker_Buck = 0;
        Bi_B_Breaker_Discharge_Boost=0;
        Bi_B_Breaker_Discharge_Buck=0;
        H1_B_Ground_Discharge=0;
        Grid_Energy_Trading_Breaker=0; %the power is sold to grid
        P1_C1=1; %the power is sold to C1

        if (V_PV_1 > V_Wind) %boosts up
        Wind_Power_Battery_Breaker_Boost=1;
        Wind_Power_Battery_Breaker_Buck=0;
        Wind_Breaker_Boost=1;
        Wind_Breaker_Buck=0;
        if (Battery_Passing_Voltage)>60
            Bi_B_Charge_Breaker_Buck=1;
            Bi_B_Charge_Breaker_Boost=0;
        elseif (Battery_Passing_Voltage<60)
            Bi_B_Charge_Breaker_Buck=0;
            Bi_B_Charge_Breaker_Boost=1;
        end

    elseif (V_PV_1 < V_Wind)
        Wind_Power_Battery_Breaker_Boost=0;
        Wind_Power_Battery_Breaker_Buck=1;
        Wind_Breaker_Boost=0;
        Wind_Breaker_Buck=1;
        
        if (Battery_Passing_Voltage)>60
            Bi_B_Charge_Breaker_Buck=1;
            Bi_B_Charge_Breaker_Boost=0;
        elseif (Battery_Passing_Voltage)<60
            Bi_B_Charge_Breaker_Buck=0;
            Bi_B_Charge_Breaker_Boost=1;
        end
        end
    end



%% CASE 3: PV and wind < Load
elseif (P_Pv + P_Wind) < (P_load) && (H1_Grid_Breaker~=0) %open (1 means open)

    % Use PV
    H1_Pv_Breaker = 1;
    H1_Grid_Circuit_Breaker = 0;
    Grid_Energy_Trading_Breaker=1;      
    Bi_B_Charge_Breaker_Buck=0; %no charging
    Bi_B_Charge_Breaker_Boost=0; %no charging
    P1_C1=0;


    if (V_PV_1)>60
        Bi_B_Breaker_Discharge_Boost=1;
        Bi_B_Breaker_Discharge_Buck=0;
        H1_B_Ground_Discharge=1;
    elseif(V_PV_1)<60
        Bi_B_Breaker_Discharge_Boost=0;
        Bi_B_Breaker_Discharge_Buck=1;
        H1_B_Ground_Discharge=1;
    end

    if (V_PV_1 > V_Wind) %boosts up
        Wind_Power_Battery_Breaker_Boost=1;
        Wind_Power_Battery_Breaker_Buck=0;
        Wind_Breaker_Boost=1;
        Wind_Breaker_Buck=0;
        
    elseif (V_PV_1 < V_Wind)
        Wind_Power_Battery_Breaker_Boost=0;
        Wind_Power_Battery_Breaker_Buck=1;
        Wind_Breaker_Boost=0;
        Wind_Breaker_Buck=1;
    end 

    
   

           
%% CASE 4:
elseif (P_Pv + P_Wind) < (P_load) && (H1_Grid_Breaker~=1) %closed (0) (no charging)

        % Use PV
    H1_Pv_Breaker = 1;
    H1_Grid_Circuit_Breaker = 0;
    Grid_Energy_Trading_Breaker=1;      
    Bi_B_Charge_Breaker_Buck=0; %(no charging)
    Bi_B_Charge_Breaker_Boost=0; %(no charging)
    Bi_B_Breaker_Discharge_Boost=0;
    Bi_B_Breaker_Discharge_Buck=0;
    H1_B_Ground_Discharge=0;
    P1_C1=0;


    if (V_PV_1 > V_Wind) %boosts up
        Wind_Power_Battery_Breaker_Boost=1;
        Wind_Power_Battery_Breaker_Buck=0;
        Wind_Breaker_Boost=1;
        Wind_Breaker_Buck=0;
        
    elseif (V_PV_1 < V_Wind)
        Wind_Power_Battery_Breaker_Boost=0;
        Wind_Power_Battery_Breaker_Buck=1;
        Wind_Breaker_Boost=0;
        Wind_Breaker_Buck=1;
    end 


%% CASE 5:
elseif (P_Pv + P_Wind+ P_Real_Grid) < P_Load 
    % Use PV
    H1_Grid_Breaker=0;
    H1_Pv_Breaker = 1;
    H1_Grid_Circuit_Breaker = 0;
    Grid_Energy_Trading_Breaker=1;      
    Bi_B_Charge_Breaker_Buck=0; %(no charging)
    Bi_B_Charge_Breaker_Boost=0; %(no charging)
    P1_C1=0;

    %discharging
    if (V_PV_1)>60
        Bi_B_Breaker_Discharge_Boost=1;
        Bi_B_Breaker_Discharge_Buck=0;
        H1_B_Ground_Discharge=1;
    elseif(V_PV_1)<60
        Bi_B_Breaker_Discharge_Boost=0;
        Bi_B_Breaker_Discharge_Buck=1;
        H1_B_Ground_Discharge=1;
    end

    if (V_PV_1 > V_Wind) %boosts up
        Wind_Power_Battery_Breaker_Boost=1;
        Wind_Power_Battery_Breaker_Buck=0;
        Wind_Breaker_Boost=1;
        Wind_Breaker_Buck=0;
        
    elseif (V_PV_1 < V_Wind) %bucks down
        Wind_Power_Battery_Breaker_Boost=0;
        Wind_Power_Battery_Breaker_Buck=1;
        Wind_Breaker_Boost=0;
        Wind_Breaker_Buck=1;
    end 

end


end

== matlab function PVHome/Subsystem5/MATLAB Function ==
  data: V_PV input; duty output; I_PV input; deltaD input
function duty = mppt_pno(V_PV, I_PV, deltaD)

persistent prevP prevDuty

if isempty(prevP)
    prevP = 0;
    prevDuty = 0.5;   % Start at 50%
end

% Current PV power
P = V_PV * I_PV;

% Basic P&O
if P > prevP
    prevDuty = prevDuty + deltaD;
else
    prevDuty = prevDuty - deltaD;
end

% Safe duty limits for boost converter
if prevDuty > 0.75
    prevDuty = 0.75;
elseif prevDuty < 0.10
    prevDuty = 0.10;
end

% Update previous power
prevP = P;

% Output duty
duty = prevDuty;

end

== matlab function PVHome/Subsystem5/MATLAB Function1 ==
  data: u input
function export_live_data(u)
% export_live_data  MATLAB Function block that writes 4 signals live into Excel
% Input: u (4-element vector)
% Exact workbook path used: 'V:\IEEE\LIVEdata.xlsx'
%
% Structure preserved: all COM/workspace actions run via evalin('base', ...)

    coder.extrinsic('evalin','assignin','actxserver','datetime','char','warning');

    persistent initialized
    if isempty(initialized)
        initialized = false;
    end

    % Convert inputs to doubles
    a = double(u(1)); b = double(u(2)); c = double(u(3)); d = double(u(4));

    % Use an .xlsx workbook for live UI updates
    excelPath = 'V:\IEEE\LIVEdata.csv';

    % Initialization block executed once (all logic runs inside evalin strings)
    if ~initialized
        % Ensure Excel COM server exists in base workspace and open/create workbook
        evalin('base', [ ...
            'if ~exist(''excelApp'',''var'') || isempty(excelApp), ' ...
                'excelApp = actxserver(''Excel.Application''); excelApp.Visible = true; ' ...
            'end; ' ...
            'if exist(''' excelPath ''',''file'')==2, ' ...
                'wb = excelApp.Workbooks.Open(''' excelPath '''); ws = wb.Worksheets.Item(1); ' ...
            'else, ' ...
                'wb = excelApp.Workbooks.Add; ws = wb.Worksheets.Item(1); ' ...
                'ws.Range(''A1'').Value = ''Timestamp''; ws.Range(''B1'').Value = ''Signal1''; ' ...
                'ws.Range(''C1'').Value = ''Signal2''; ws.Range(''D1'').Value = ''Signal3''; ' ...
                'ws.Range(''E1'').Value = ''Signal4''; wb.SaveAs(''' excelPath '''); ' ...
            'end; ' ...
            'if ~exist(''excelRow'',''var'') || isempty(excelRow), ur = ws.UsedRange; excelRow = double(ur.Rows.Count) + 1; end;']);

        initialized = true;
    end

    % Create timestamp string using datetime (host MATLAB)
    ts = char(datetime('now', 'Format', 'yyyy-MM-dd HH:mm:ss.SSS'));

    % Pass values into base workspace temporary variables (RHS only)
    assignin('base', 'tmp_ts', ts);
    assignin('base', 'tmp_a', a);
    assignin('base', 'tmp_b', b);
    assignin('base', 'tmp_c', c);
    assignin('base', 'tmp_d', d);

    % Perform the worksheet write and force Excel UI update (all inside evalin)
    % Note: r is the row written; we save, increment excelRow, then force repaint and scroll.
    evalin('base', [ ...
        'r = excelRow; ' ...
        'ws.Range([''A'' num2str(r)]).Value = tmp_ts; ' ...
        'ws.Range([''B'' num2str(r)]).Value = tmp_a; ' ...
        'ws.Range([''C'' num2str(r)]).Value = tmp_b; ' ...
        'ws.Range([''D'' num2str(r)]).Value = tmp_c; ' ...
        'ws.Range([''E'' num2str(r)]).Value = tmp_d; ' ...
        'wb.Save; ' ...
        'excelRow = r + 1; ' ...
        'try, excelApp.ScreenUpdating = true; excelApp.Calculate; ' ...
             'if ~isempty(excelApp.ActiveWindow), excelApp.ActiveWindow.ScrollRow = r; end; ' ...
             'pause(0.02); ' ...
        'end;']);

end

== matlab function PVHome/Subsystem2/MATLAB Function2 ==
  data: x input; a output; ma input; shift_k input; b output; c output
function [a,b,c]=ref_generation(x,ma,shift_k)
a=(ma*(sin((x)+shift_k)));
b=(ma*(sin((x)+shift_k-(2*pi/3))));
c=(ma*(sin((x)+shift_k+(2*pi/3))));

%ma is modulation index
%x is wt rad/s
%shift_k is phase angle

== matlab function PVHome/Subsystem2/MATLAB Function3 ==
  data: u input; y output
function y = fcn(u)
% This will output 1 - u
y = 1 - u;

== matlab function PVHome/Subsystem5/MATLAB Function2 ==
  data: x input; a output; ma input; shift_k input; b output; c output
function [a,b,c]=ref_generation(x,ma,shift_k)
a=(ma*(sin((x)+shift_k)));
b=(ma*(sin((x)+shift_k-(2*pi/3))));
c=(ma*(sin((x)+shift_k+(2*pi/3))));

%ma is modulation index
%x is wt rad/s
%shift_k is phase angle

== matlab function PVHome/Subsystem5/MATLAB Function3 ==
  data: u input; y output
function y = fcn(u)
% This will output 1 - u
y = 1 - u;

== matlab function PVHome/Subsystem5/MATLAB Function4 ==
  data: u input; y output
function y = fcn(u)
% This will output 1 - u
y = 1 - u;

== matlab function PVHome/Subsystem5/MATLAB Function6 ==
  data: u input; y output
function y = fcn(u)
% This will output 1 - u
y = 1 - u;

== matlab function PVHome/Subsystem5/MATLAB Function7 ==
  data: V_PV_1 input; Wind_Breaker_Boost_Signal_Out output; V_Wind input
function Wind_Breaker_Boost_Signal_Out = fcn(V_PV_1, V_Wind)
V_PV_1 = abs(V_PV_1);
V_Wind = abs(V_Wind);

D=1-(V_PV_1/V_Wind);
Wind_Breaker_Boost_Signal_Out = D; %Vout

== matlab function PVHome/Subsystem5/MATLAB Function8 ==
  data: Sixty input; Wind_Breaker_Boost_Signal_Out output; V_PV_1 input
function Wind_Breaker_Boost_Signal_Out = fcn(Sixty, V_PV_1)
Sixty = abs(Sixty);
V_PV_1 = abs(V_PV_1);

D=1-(Sixty/V_PV_1);
Wind_Breaker_Boost_Signal_Out = D; %Vout
